simulink model "model_regulator"  (R2024a)
settings: Solver=FixedStepAuto  StartTime=0.0  StopTime=10.0  FixedStep=0.001  RelTol=1e-3
undefined symbols (not defined in the file): k0, k1
settings Model: Creator=main  LastModifiedBy=main

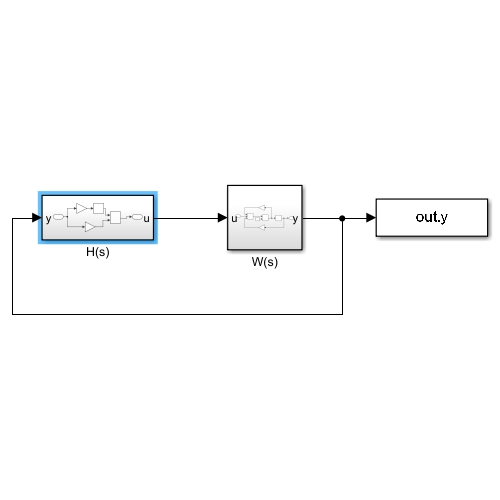
[thumbnail: Simulink's stored preview of the top-level diagram]
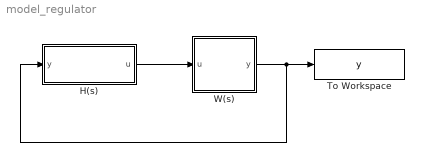
== system model_regulator ==
  H(s) : Subsystem
  To Workspace : ToWorkspace  VariableName=y  SaveFormat=Timeseries  SampleTime=-1
  W(s) : Subsystem
  wires:
  W(s)/1(y) -> H(s)/1(y), To Workspace/1
  H(s)/1(u) -> W(s)/1(u)

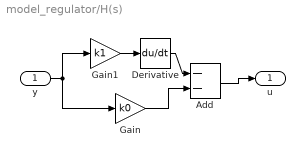
== system model_regulator/H(s) ==
  y : Inport
  Add : Sum  Inputs=--
  Derivative : Derivative
  Gain : Gain  Gain=k0
  Gain1 : Gain  Gain=k1
  u : Outport
  wires:
  y/1 -> Gain/1, Gain1/1
  Add/1 -> u/1
  Derivative/1 -> Add/1
  Gain1/1 -> Derivative/1
  Gain/1 -> Add/2

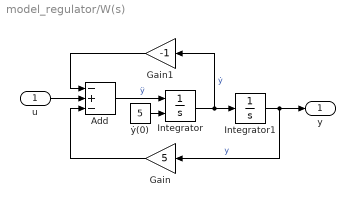
== system model_regulator/W(s) ==
  u : Inport
  Add : Sum  Inputs=-+-
  Gain : Gain  Gain=5
  Gain1 : Gain  Gain=-1
  Integrator : Integrator  InitialConditionSource=external  InitialCondition=5
  Integrator1 : Integrator
  ẏ(0) : Constant  Value=5
  y : Outport
  wires:
  Integrator1/1 -> y/1, Gain/1  "y"
  Add/1 -> Integrator/1  "ÿ"
  Gain/1 -> Add/3
  Integrator/1 -> Gain1/1, Integrator1/1  "ẏ"
  Gain1/1 -> Add/1
  ẏ(0)/1 -> Integrator/2
  u/1 -> Add/2
